simulink model "LPV_Nonlinear_Simulation_16b"  (R2016b)
settings: Solver=ode3  StartTime=0.0  StopTime=100  FixedStep=ts  RelTol=1e-3
InitFcn:
  | InitGyro
values from neighbouring files (symbols this model uses):
  ts = 0.01    [InitGyro.m]    (also in Parameters.m)
undefined symbols (not defined in the file): sys
libraries: simulink x2, simulink_extras x1, cstblocks x1
settings Model: Creator=jt  LastModifiedBy=c00rts28
settings DataIOCC: LimitDataPoints=on  SaveFormat=Array
settings OptimizationCC: BlockReduction=off  BooleanDataType=off  LifeSpan=inf
settings DebuggingCC: SaveWithParameterizedLinksMsg=none  UnderspecifiedInitializationDetection=Classic  MergeDetectMultiDrivingBlocksExec=none  SignalResolutionControl=TryResolveAllWithWarning  SFUnexpectedBacktrackingDiag=warning  SFNoUnconditionalDefaultTransitionDiag=warning  SFExecutionAtInitializationDiag=none
settings HardwareCC: ProdBitPerPointer=32  ProdBitPerSizeT=32  ProdBitPerPtrDiffT=32  ProdLargestAtomicFloat=None  ProdWordSize=32  ProdHWDeviceType=Generic->32-bit x86 compatible  TargetBitPerPointer=64  TargetBitPerSizeT=64  TargetBitPerPtrDiffT=64  TargetLongLongMode=on  TargetIntDivRoundTo=Zero  TargetEndianess=LittleEndian  TargetWordSize=64  TargetHWDeviceType=MATLAB Host  ProdEqTarget=off
settings ModelReferenceCC: PropagateSignalLabelsOutOfModel=off
settings RTWCC: RTWCompilerOptimization=on
settings CodeAppCC: MaxIdLength=95
settings GRTTargetCC: TargetLangStandard=C89/C90 (ANSI)  GeneratePreprocessorConditionals=Disable all
settings ConfigComp: CovMetricSettings=dw  CovHtmlReporting=on  CovSaveCumulativeToWorkspaceVar=on  CovSaveSingleToWorkspaceVar=on  CovExternalEMLEnable=off  CovSFcnEnable=off

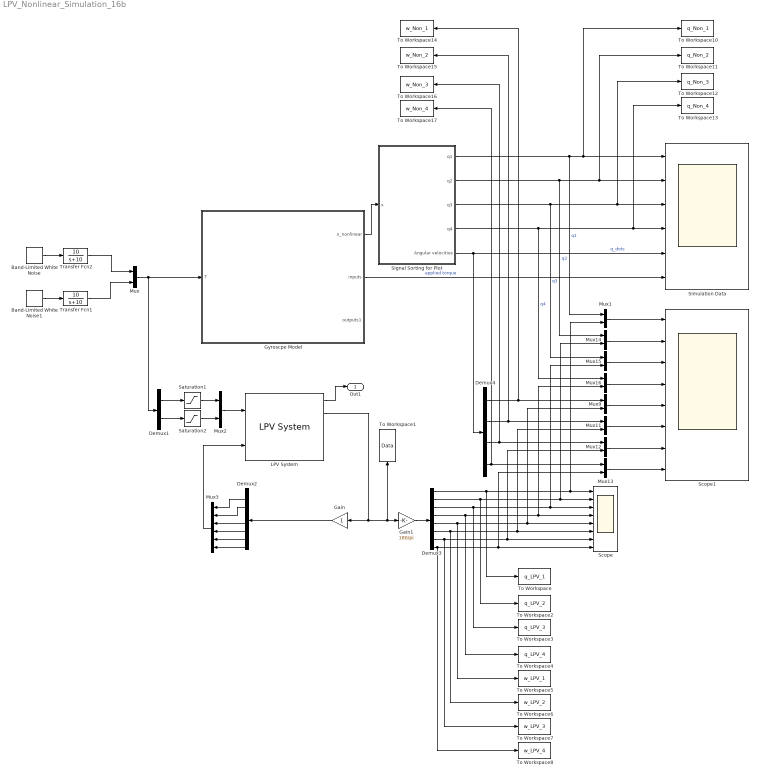
== system LPV_Nonlinear_Simulation_16b ==
  Band-Limited White Noise : simulink/Sources/Band-Limited White Noise  Cov=[0.000000001]  Ts=ts  seed=[23341]
  Band-Limited White Noise1 : simulink/Sources/Band-Limited White Noise  Cov=[0.000000001]  Ts=ts  seed=[23341]
  Demux1 : Demux  Outputs=2
  Demux2 : Demux  Outputs=8
  Demux3 : Demux  Outputs=8
  Demux4 : Demux
  Gain : Gain
  Gain1 : Gain  Gain=180/pi
  Gyroscpe Model : Subsystem
  LPV System : cstblocks/LPV System  sys=sysLPV  x0=[-0.21 -0.21 0.09 0.35 -0.55 0.55 0.45 0.45]';  uOffset=0  yOffset=0  xOffset=0  opEquilOption=off  dxOffset=0  sysFixedOption=Use the first model in state-space array  sysFixed=[]  AFixed=0  BFixed=0  CFixed=0  DFixed=0  uDelayFixed=true  yDelayFixed=true  iDelayFixed=true  IMethod=Linear  EMethod=Clip  IndexSearch=Binary search  IndexBegin=on  OutputX=on  OutputXdot=on  OutputLTI=on  OutputOP=on  DataType=double  SimMode=Interpreted execution  InitBufferSize=1024  FixedBuffer=off
  Mux{,1..2,9,11..16} (10 alike) : Mux  Inputs=2
  Mux3 : Mux  Inputs=6
  Saturation1 : Saturate  UpperLimit=0.666  LowerLimit=-0.666
  Saturation2 : Saturate  UpperLimit=2.44  LowerLimit=-2.44
  Scope : Scope  NumInputPorts=8
  Scope1 : Scope  NumInputPorts=8
  Signal Sorting for Plot : Subsystem
  Simulation Data : Scope  NumInputPorts=6
  To Workspace : ToWorkspace  VariableName=q_LPV_1  SaveFormat=Timeseries  SampleTime=-1
  To Workspace1 : ToWorkspace  VariableName=Data  SaveFormat=Timeseries  SampleTime=-1
  To Workspace10 : ToWorkspace  VariableName=q_Non_1  SaveFormat=Timeseries  SampleTime=-1
  To Workspace11 : ToWorkspace  VariableName=q_Non_2  SaveFormat=Timeseries  SampleTime=-1
  To Workspace12 : ToWorkspace  VariableName=q_Non_3  SaveFormat=Timeseries  SampleTime=-1
  To Workspace13 : ToWorkspace  VariableName=q_Non_4  SaveFormat=Timeseries  SampleTime=-1
  To Workspace14 : ToWorkspace  VariableName=w_Non_1  SaveFormat=Timeseries  SampleTime=-1
  To Workspace15 : ToWorkspace  VariableName=w_Non_2  SaveFormat=Timeseries  SampleTime=-1
  To Workspace16 : ToWorkspace  VariableName=w_Non_3  SaveFormat=Timeseries  SampleTime=-1
  To Workspace17 : ToWorkspace  VariableName=w_Non_4  SaveFormat=Timeseries  SampleTime=-1
  To Workspace2 : ToWorkspace  VariableName=q_LPV_2  SaveFormat=Timeseries  SampleTime=-1
  To Workspace3 : ToWorkspace  VariableName=q_LPV_3  SaveFormat=Timeseries  SampleTime=-1
  To Workspace4 : ToWorkspace  VariableName=q_LPV_4  SaveFormat=Timeseries  SampleTime=-1
  To Workspace5 : ToWorkspace  VariableName=w_LPV_1  SaveFormat=Timeseries  SampleTime=-1
  To Workspace6 : ToWorkspace  VariableName=w_LPV_2  SaveFormat=Timeseries  SampleTime=-1
  To Workspace7 : ToWorkspace  VariableName=w_LPV_3  SaveFormat=Timeseries  SampleTime=-1
  To Workspace8 : ToWorkspace  VariableName=w_LPV_4  SaveFormat=Timeseries  SampleTime=-1
  Transfer Fcn1 : TransferFcn  Numerator=[10]  Denominator=[1 10]
  Transfer Fcn2 : TransferFcn  Numerator=[10]  Denominator=[1 10]
  Out1 : Outport
  wires:
  Gyroscpe Model/1(x_nonlinear) -> Signal Sorting for Plot/1(x)
  Signal Sorting for Plot/1(q1) -> To Workspace10/1, Simulation Data/1, Mux1/1  "q1"
  Signal Sorting for Plot/2(q2) -> To Workspace11/1, Simulation Data/2, Mux14/1  "q2"
  Signal Sorting for Plot/4(q4) -> Simulation Data/4, To Workspace13/1, Mux16/1  "q4"
  Signal Sorting for Plot/3(q3) -> Simulation Data/3, To Workspace12/1, Mux15/1  "q3"
  Gyroscpe Model/2(inputs) -> Simulation Data/6  "applied torque"
  LPV System/1 -> Out1/1
  Mux3/1 -> LPV System/2
  Demux1/1 -> Saturation1/1
  Saturation1/1 -> Mux2/1
  Saturation2/1 -> Mux2/2
  Demux1/2 -> Saturation2/1
  Gain/1 -> Demux2/1
  Demux2/8 -> Mux3/6
  Demux2/7 -> Mux3/5
  Demux2/6 -> Mux3/4
  Demux2/5 -> Mux3/3
  Demux2/2 -> Mux3/1
  Demux2/3 -> Mux3/2
  Demux3/1 -> Scope/1, Mux1/2, To Workspace/1
  Demux3/2 -> Scope/2, Mux14/2, To Workspace2/1
  Demux3/3 -> Scope/3, Mux15/2, To Workspace3/1
  Demux3/4 -> Scope/4, Mux16/2, To Workspace4/1
  Demux3/5 -> Scope/5, Mux9/2, To Workspace5/1
  Demux3/6 -> Scope/6, Mux11/2, To Workspace6/1
  Demux3/7 -> Scope/7, Mux12/2, To Workspace7/1
  Demux3/8 -> Scope/8, Mux13/2, To Workspace8/1
  Mux9/1 -> Scope1/5
  Mux12/1 -> Scope1/7
  Mux13/1 -> Scope1/8
  Signal Sorting for Plot/5(Angular velocities) -> Simulation Data/5, Demux4/1  "q_dots"
  Demux4/1 -> To Workspace14/1, Mux9/1
  Demux4/2 -> To Workspace15/1, Mux11/1
  Demux4/3 -> To Workspace16/1, Mux12/1
  Demux4/4 -> To Workspace17/1, Mux13/1
  Mux1/1 -> Scope1/1
  Mux14/1 -> Scope1/2
  Mux15/1 -> Scope1/3
  Mux16/1 -> Scope1/4
  Mux2/1 -> LPV System/1
  Mux/1 -> Demux1/1, Gyroscpe Model/1(T)
  LPV System/2 -> Gain1/1, To Workspace1/1, Gain/1
  Band-Limited White Noise/1 -> Transfer Fcn2/1
  Band-Limited White Noise1/1 -> Transfer Fcn1/1
  Mux11/1 -> Scope1/6
  Gain1/1 -> Demux3/1
  Transfer Fcn1/1 -> Mux/2
  Transfer Fcn2/1 -> Mux/1

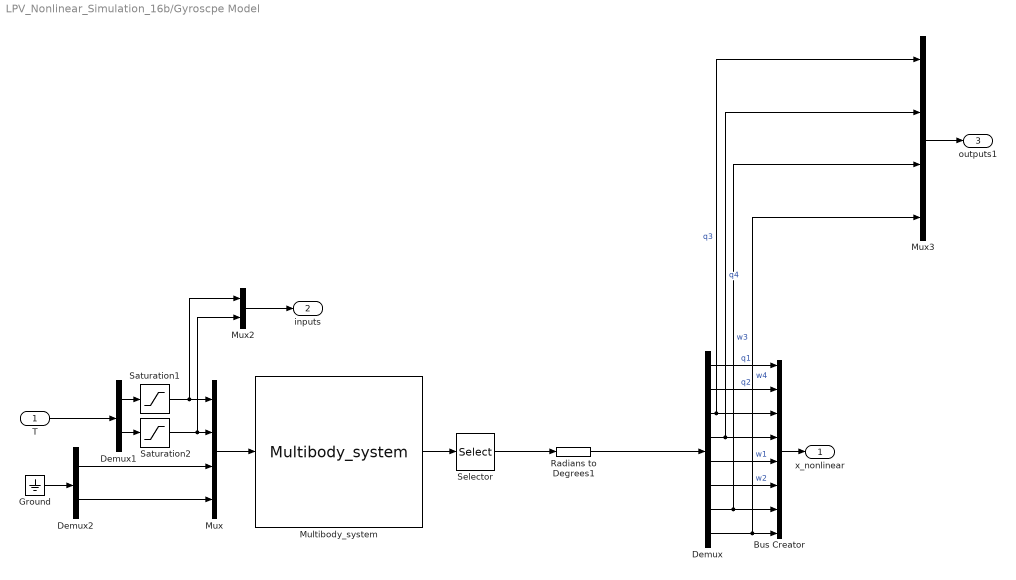
== system LPV_Nonlinear_Simulation_16b/Gyroscpe Model ==
  T : Inport
  Bus Creator : BusCreator  Inputs=8
  Demux : Demux  Outputs=8
  Demux1 : Demux  Outputs=2
  Demux2 : Demux  Outputs=2
  Ground : Ground
  Multibody_system : S-Function  FunctionName=Multibody_system  Parameters=paraStruct, initY, initDy  SFunctionDeploymentMode=off  EnableBusSupport=off  mask(Neweul-M2 nonlinear model){paraStruct=sys.parameters.data, initY=[-0.21 -0.21 0.09 0.35]';, initDy=[-0.55 0.55 0.45 0.45]';}
      mask prompts: paraStruct "Neweul-M2 Parameter Structure"; initY "Initial coordinates"; initDy "Initial velocities"
      mask help:
      | State-state representation of a multibody system
      | created with Neueul-MÂ².
      |
      | In order to run a simulation in Simulink you have to provide
      | the following input parameters:
      |   * Neweul-M2 Parameter Structure (sys.parameters.data)
      |     ... Structure containing all user-defined parameters
      |   * Initial coordinates (zeros(sys.counters.genCoord,1))
      |     ... Initial values for the generalized coordinates
      |   * Initial velocities (zeros(sys.dof,1))
      |     ... Initial values for the generalized velocities
      |
      | Neweul-MÂ²
      | Multibody systems based on symbolic Newton-Euler-Equations
      | Copyright (c) ITM University of Stuttgart, www.itm.uni-stuttgart.de
      mask Display:
      | port_label('output',1,'states [8x1]');
      | port_label('input',1,'control [4x1]');
  Mux : Mux
  Mux2 : Mux  Inputs=2
  Mux3 : Mux
  Radians to Degrees1 : simulink_extras/Transformations/Radians to Degrees
  Saturation1 : Saturate  UpperLimit=0.666  LowerLimit=-0.666
  Saturation2 : Saturate  UpperLimit=2.44  LowerLimit=-2.44
  Selector : Selector  IndexOptions=Index vector (dialog)  Indices=1:8  OutputSizes=1
  x_nonlinear : Outport
  inputs : Outport  Port=2
  outputs1 : Outport  Port=3
  wires:
  Multibody_system/1 -> Selector/1
  Selector/1 -> Radians to Degrees1/1
  Bus Creator/1 -> x_nonlinear/1
  Mux/1 -> Multibody_system/1
  Demux2/2 -> Mux/4
  Demux2/1 -> Mux/3
  Demux1/2 -> Saturation2/1
  Mux2/1 -> inputs/1
  Saturation2/1 -> Mux2/2, Mux/2
  Saturation1/1 -> Mux2/1, Mux/1
  Demux1/1 -> Saturation1/1
  T/1 -> Demux1/1
  Ground/1 -> Demux2/1
  Mux3/1 -> outputs1/1
  Demux/1 -> Bus Creator/1  "q1"
  Demux/2 -> Bus Creator/2  "q2"
  Demux/3 -> Mux3/1, Bus Creator/3  "q3"
  Demux/5 -> Bus Creator/5  "w1"
  Demux/4 -> Mux3/2, Bus Creator/4  "q4"
  Demux/6 -> Bus Creator/6  "w2"
  Demux/8 -> Mux3/4, Bus Creator/8  "w4"
  Demux/7 -> Mux3/3, Bus Creator/7  "w3"
  Radians to Degrees1/1 -> Demux/1

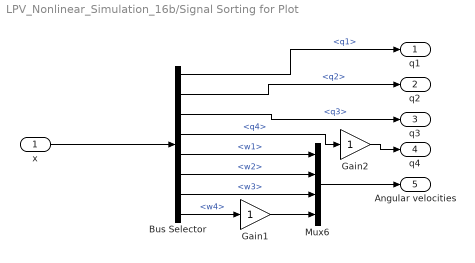
== system LPV_Nonlinear_Simulation_16b/Signal Sorting for Plot ==
  x : Inport
  Bus Selector : BusSelector  OutputSignals=q1,q2,q3,q4,w1,w2,w3,w4
  Gain1 : Gain
  Gain2 : Gain
  Mux6 : Mux
  q1 : Outport
  q2 : Outport  Port=2
  q3 : Outport  Port=3
  q4 : Outport  Port=4
  Angular velocities : Outport  Port=5
  wires:
  Bus Selector/3 -> q3/1  "<q3>"
  Bus Selector/2 -> q2/1  "<q2>"
  Bus Selector/1 -> q1/1  "<q1>"
  Mux6/1 -> Angular velocities/1
  Bus Selector/5 -> Mux6/1  "<w1>"
  Bus Selector/6 -> Mux6/2  "<w2>"
  Bus Selector/7 -> Mux6/3  "<w3>"
  x/1 -> Bus Selector/1
  Bus Selector/8 -> Gain1/1  "<w4>"
  Gain1/1 -> Mux6/4
  Bus Selector/4 -> Gain2/1  "<q4>"
  Gain2/1 -> q4/1
